simulink subsystem "Mission_Manager_Interface"  (R2025b)
settings: Solver=VariableStepAuto  StartTime=0.0  StopTime=10.0  RelTol=1e-3
undefined symbols (not defined in the file or in its folder): dt_control
libraries: ros2lib x2
settings Model: Creator=kjhaydon  LastModifiedBy=kjhaydon

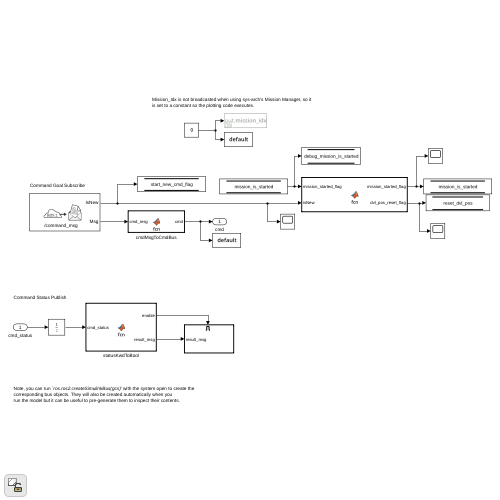
[thumbnail: Simulink's stored preview of the top-level diagram]
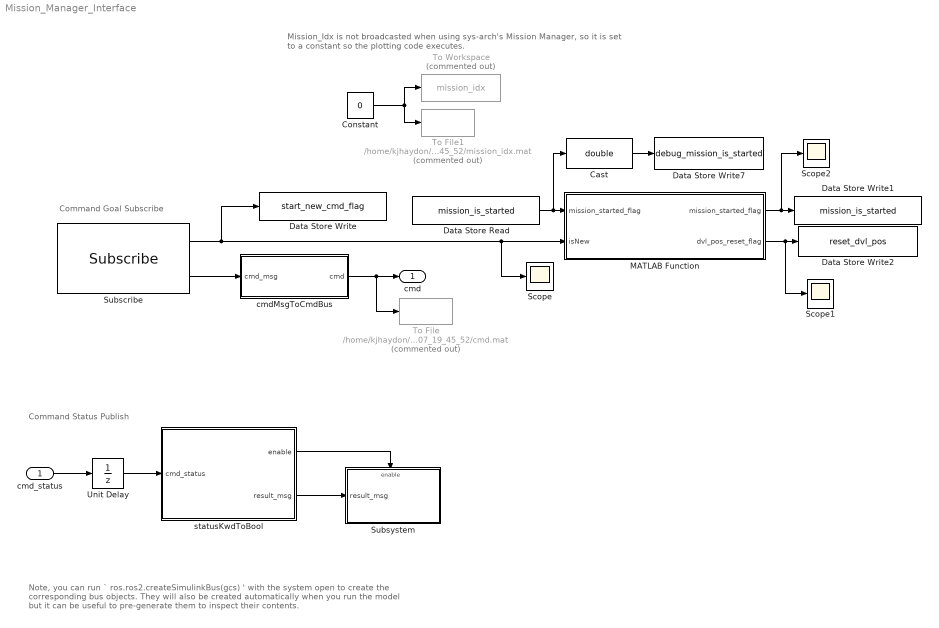
== system Mission_Manager_Interface ==
  note: Note, you can run ` ros.ros2.createSimulinkBus(gcs) ' with the system open to create the
      | corresponding bus objects. They will also be created automatically when you
      | run the model but it can be useful to pre-generate them to inspect their contents.
  note: Command Status Publish
  note: Command Goal Subscribe
  note: Mission_Idx is not broadcasted when using sys-arch's Mission Manager, so it
      | is set to a constant so the plotting code executes.
  cmd_status : Inport  SampleTime=dt_control
  Cast : DataTypeConversion  OutDataTypeStr=double  SaturateOnIntegerOverflow=off  RndMeth=Floor
  Constant : Constant  Value=0
  Data Store Read : DataStoreRead  DataStoreName=mission_is_started  IndexOptions=Index vector (dialog)  Indices=1  OutputSizes=1
  Data Store Write : DataStoreWrite  DataStoreName=start_new_cmd_flag  SampleTime=dt_control  IndexOptions=Index vector (dialog)  Indices=1  OutputSizes=1
  Data Store Write1 : DataStoreWrite  DataStoreName=mission_is_started  IndexOptions=Index vector (dialog)  Indices=1  OutputSizes=1
  Data Store Write2 : DataStoreWrite  DataStoreName=reset_dvl_pos  IndexOptions=Index vector (dialog)  Indices=1  OutputSizes=1
  Data Store Write7 : DataStoreWrite  DataStoreName=debug_mission_is_started  IndexOptions=Index vector (dialog)  Indices=1  OutputSizes=1
  MATLAB Function : MATLAB Function  TreatAsAtomicUnit=on
  Scope : Scope
      settings: ActiveDisplayYMinimum=-1  ActiveDisplayYMaximum=1  DataLoggingVariableName=ScopeData4
  Scope1 : Scope
      settings: ActiveDisplayYMinimum=-1  ActiveDisplayYMaximum=1  DataLoggingVariableName=ScopeData7
  Scope2 : Scope
      settings: ActiveDisplayYMinimum=-0.12499999999999997  ActiveDisplayYMaximum=1.125  DataLoggingVariableName=ScopeData5
  Subscribe : ros2lib/Subscribe  topicSource=Specify your own  topic=/command_msg  messageType=custom_interfaces/Goal  sampleTime=0.01  QOSHistory=Keep last  QOSDepth=10  QOSReliability=Reliable  QOSDurability=Volatile  QOSDeadline=Inf  QOSLifespan=Inf  QOSLiveliness=Automatic  QOSLeaseDuration=Inf  QOSAvoidROSNamespaceConventions=off
  Subsystem : Subsystem
  To File : ToFile  Commented=on  Filename=/home/kjhaydon/Github/Robosub/SimulinkPlant/data/2026_07_07_19_45_52/cmd.mat  MatrixName=cmd  SaveFormat=Timeseries
  To File1 : ToFile  Commented=on  Filename=/home/kjhaydon/Github/Robosub/SimulinkPlant/data/2026_07_07_19_45_52/mission_idx.mat  MatrixName=mission_idx  SaveFormat=Timeseries
  To Workspace : ToWorkspace  Commented=on  VariableName=mission_idx  SaveFormat=Timeseries  SampleTime=dt_control
  Unit Delay : UnitDelay  SampleTime=-1  HasFrameUpgradeWarning=on
  cmdMsgToCmdBus : MATLAB Function  TreatAsAtomicUnit=on
  statusKwdToBool : MATLAB Function  TreatAsAtomicUnit=on
  cmd : Outport  SampleTime=dt_control
  wires:
  cmd_status/1 -> Unit Delay/1
  statusKwdToBool/1(enable) -> Subsystem/Enable
  Unit Delay/1 -> statusKwdToBool/1(cmd_status)
  statusKwdToBool/2(result_msg) -> Subsystem/1(result_msg)
  Subscribe/1 -> Data Store Write/1, Scope/1, MATLAB Function/2(isNew)
  Subscribe/2 -> cmdMsgToCmdBus/1(cmd_msg)
  cmdMsgToCmdBus/1(cmd) -> To File/1, cmd/1
  Constant/1 -> To Workspace/1, To File1/1
  MATLAB Function/1(mission_started_flag) -> Data Store Write1/1, Scope2/1
  MATLAB Function/2(dvl_pos_reset_flag) -> Data Store Write2/1, Scope1/1
  Data Store Read/1 -> MATLAB Function/1("mission_started_flag "), Cast/1
  Cast/1 -> Data Store Write7/1

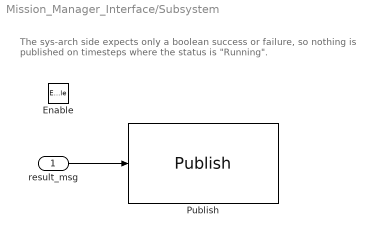
== system Mission_Manager_Interface/Subsystem ==
  note: The sys-arch side expects only a boolean success or failure, so nothing
      | is published on timesteps where the status is "Running".
  result_msg : Inport
  Enable : EnablePort
  Publish : ros2lib/Publish  topicSource=Specify your own  topic=/command_result  messageType=custom_interfaces/Result  QOSHistory=Keep last  QOSDepth=10  QOSReliability=Reliable  QOSDurability=Volatile  QOSDeadline=Inf  QOSLifespan=Inf  QOSLiveliness=Automatic  QOSLeaseDuration=Inf  QOSAvoidROSNamespaceConventions=off
  wires:
  result_msg/1 -> Publish/1

== matlab function Mission_Manager_Interface/MATLAB Function ==
  data: mission_started_flag output; dvl_pos_reset_flag output; mission_started_flag input; isNew input
function [mission_started_flag, dvl_pos_reset_flag]  = fcn(mission_started_flag, isNew)

if(~mission_started_flag && isNew)
    dvl_pos_reset_flag = true;
    mission_started_flag = true;
elseif(mission_started_flag)
    dvl_pos_reset_flag = false;
else
    dvl_pos_reset_flag = false;
end

== matlab function Mission_Manager_Interface/cmdMsgToCmdBus ==
  data: cmd_msg input Bus: SL_Bus_custom_interfaces_Goal; cmd output Bus: cmd_bus
function cmd = fcn(cmd_msg)

cmd = cmdMsgToCmdBus(cmd_msg);

end

== matlab function Mission_Manager_Interface/statusKwdToBool ==
  data: enable output; cmd_status input; result_msg output Bus: SL_Bus_custom_interfaces_Result
function [enable, result_msg]   = fcn(cmd_status)

[enable, result_msg] = statusKwdToBool(cmd_status);
